simulink model "untitled"  (R2025b)
settings: Solver=FixedStepAuto  StartTime=0.0  StopTime=20  FixedStep=0.001  RelTol=1e-3
libraries: simulink x2, slpidlib x2
settings Model: Creator=Utente  LastModifiedBy=zinga

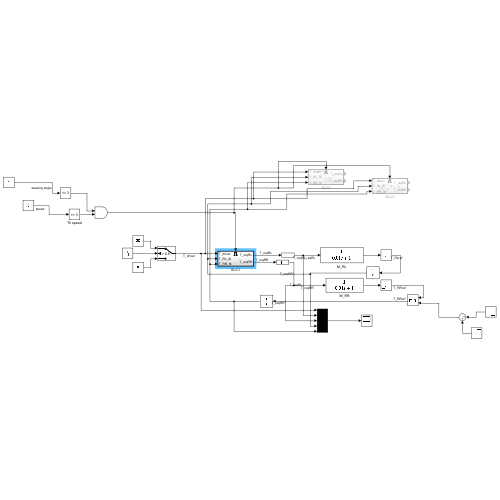
[thumbnail: Simulink's stored preview of the top-level diagram]
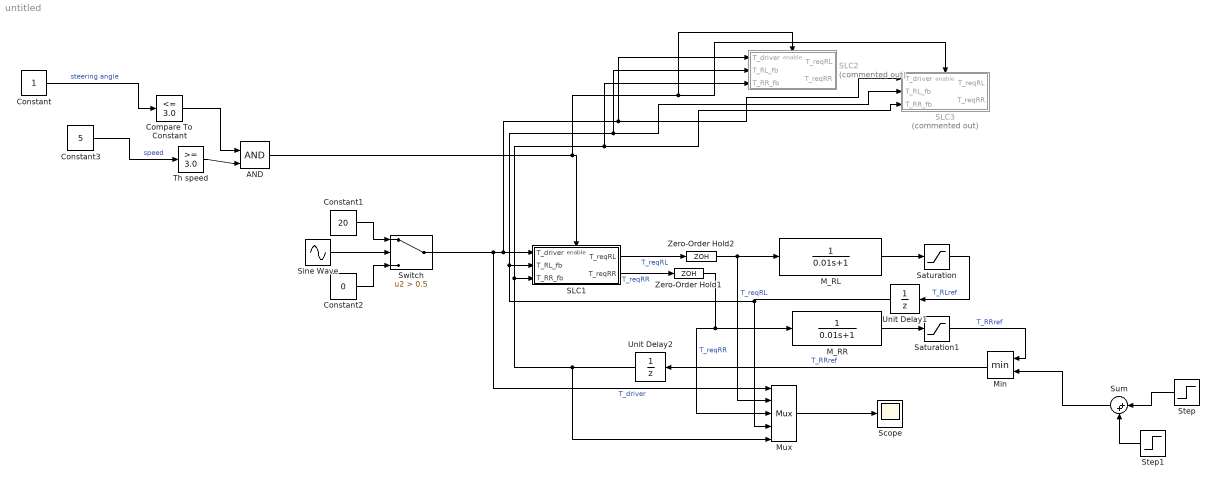
== system untitled ==
  AND : Logic  IconShape=distinctive  AllPortsSameDT=off  OutDataTypeStr=boolean
  Compare To Constant : simulink/Logic and Bit Operations/Compare To Constant  relop=<=  const=3.0  OutDataTypeStr=boolean
  Constant : Constant
  Constant1 : Constant  Value=20
  Constant2 : Constant  Value=0
  Constant3 : Constant  Value=5
  M_RL : TransferFcn  Denominator=[0.01 1]
  M_RR : TransferFcn  Denominator=[0.01 1]
  Min : MinMax  Inputs=2
  Mux : Mux  Inputs=5
  SLC1 : Subsystem  TreatAsAtomicUnit=on
  SLC2 : Subsystem  Commented=on  TreatAsAtomicUnit=on
  SLC3 : Subsystem  Commented=on  TreatAsAtomicUnit=on
  Saturation : Saturate  UpperLimit=21  LowerLimit=-21
  Saturation1 : Saturate  UpperLimit=21  LowerLimit=-21
  Scope : Scope
      settings: ActiveDisplayYMinimum=1.4080718802065189  ActiveDisplayYMaximum=18.911191161536266
  Sine Wave : Sin  Frequency=0.2  SampleTime=0.01
  Step : Step  Time=3  Before=21  After=8  SampleTime=0
  Step1 : Step  Time=9  After=13  SampleTime=0
  Sum : Sum  Inputs=|++
  Switch : Switch  Criteria=u2 > Threshold  Threshold=0.5  SaturateOnIntegerOverflow=off  InputSameDT=off
  Th speed : simulink/Logic and Bit Operations/Compare To Constant  relop=>=  const=3.0  OutDataTypeStr=boolean
  Unit Delay1 : UnitDelay  SampleTime=-1  HasFrameUpgradeWarning=on
  Unit Delay2 : UnitDelay  SampleTime=-1  HasFrameUpgradeWarning=on
  Zero-Order Hold1 : ZeroOrderHold  SampleTime=0.01
  Zero-Order Hold2 : ZeroOrderHold  SampleTime=0.01
  wires:
  Compare To Constant/1 -> AND/1
  Constant/1 -> Compare To Constant/1  "steering angle"
  SLC1/1(T_reqRL) -> Zero-Order Hold2/1  "T_reqRL"
  SLC1/2(T_reqRR) -> Zero-Order Hold1/1  "T_reqRR"
  Mux/1 -> Scope/1
  M_RL/1 -> Saturation/1
  Saturation/1 -> Unit Delay1/1  "T_RLref"
  Sine Wave/1 -> Switch/2
  Constant1/1 -> Switch/1
  Constant2/1 -> Switch/3
  Switch/1 -> Mux/1, SLC3/1(T_driver), SLC2/1(T_driver), SLC1/1(T_driver)  "T_driver"
  M_RR/1 -> Saturation1/1
  Min/1 -> Unit Delay2/1  "T_RRref"
  Constant3/1 -> Th speed/1  "speed"
  Th speed/1 -> AND/2
  AND/1 -> SLC1/Enable, SLC3/Enable, SLC2/Enable
  Saturation1/1 -> Min/1  "T_RRref"
  Step/1 -> Sum/1
  Sum/1 -> Min/2
  Step1/1 -> Sum/2
  Unit Delay1/1 -> Mux/4, SLC1/2(T_RL_fb), SLC3/2(T_RL_fb), SLC2/2(T_RL_fb)
  Unit Delay2/1 -> SLC2/3(T_RR_fb), SLC3/3(T_RR_fb), SLC1/3(T_RR_fb), Mux/5
  Zero-Order Hold1/1 -> Mux/3, M_RR/1  "T_reqRR"
  Zero-Order Hold2/1 -> Mux/2, M_RL/1  "T_reqRL"

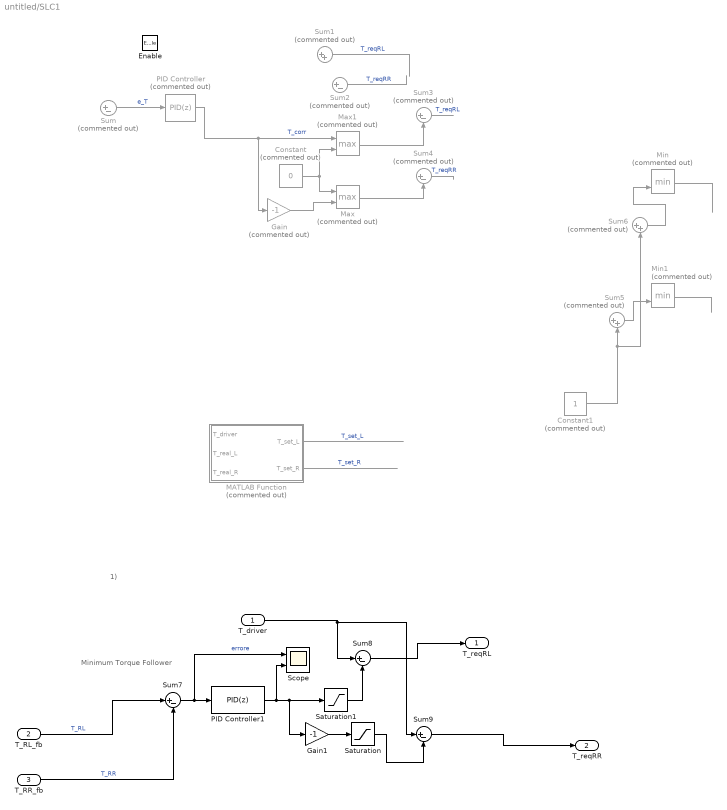
== system untitled/SLC1 ==
  note: Minimum Torque Follower
  note: 1)
  T_driver : Inport
  T_RL_fb : Inport  Port=2
  T_RR_fb : Inport  Port=3
  Enable : EnablePort
  Constant : Constant  Commented=on  Value=0
  Constant1 : Constant  Commented=on
  Gain : Gain  Commented=on  Gain=-1
  Gain1 : Gain  Gain=-1
  MATLAB Function : MATLAB Function  Commented=on  TreatAsAtomicUnit=on
  Max : MinMax  Commented=on  Function=max  Inputs=2
  Max1 : MinMax  Commented=on  Function=max  Inputs=2
  Min : MinMax  Commented=on  Inputs=2
  Min1 : MinMax  Commented=on  Inputs=2
  PID Controller : slpidlib/PID Controller  Commented=on  Controller=PID  Form=Parallel  TimeDomain=Discrete-time  UseExternalTs=off  SampleTime=0.05  IntegratorMethod=Forward Euler  FilterMethod=Forward Euler  ControllerParametersSource=internal  P=0.02  I=5  UseKiTs=off  D=0  UseExternalDerivativeSource=off  N=100  UseFilter=on  TunerSelectOption=Transfer Function Based (PID Tuner App)  InitialConditionSource=internal  InitialConditionForIntegrator=0  InitialConditionForFilter=0  DifferentiatorICPrevScaledInput=0  ExternalReset=none  TrackingMode=off  Kt=1  LimitOutput=on  SatLimitsSource=internal  UpperSaturationLimit=21  LowerSaturationLimit=-21  LinearizeAsGain=on  AntiWindupMode=clamping  Kb=1  LimitIntegrator=off  UpperIntegratorSaturationLimit=inf  LowerIntegratorSaturationLimit=-inf  POutMin=[]  POutMax=[]  IOutMin=[]  IOutMax=[]  DOutMin=[]  DOutMax=[]  NOutMin=[]  NOutMax=[]  SumOutMin=[]  SumOutMax=[]  SaturationOutMin=[]  SaturationOutMax=[]  PParamMin=[]  PParamMax=[]  IParamMin=[]  IParamMax=[]  DParamMin=[]  DParamMax=[]  NParamMin=[]  NParamMax=[]  KbParamMin=[]  KbParamMax=[]  KtParamMin=[]  KtParamMax=[]  KbOutMin=[]  KbOutMax=[]  KtOutMin=[]  KtOutMax=[]  IntegratorOutMin=[]  IntegratorOutMax=[]  FilterOutMin=[]  FilterOutMax=[]  SumI1OutMin=[]  SumI1OutMax=[]  SumI2OutMin=[]  SumI2OutMax=[]  SumI3OutMin=[]  SumI3OutMax=[]  SumI4OutMin=[]  SumI4OutMax=[]  SumDOutMin=[]  SumDOutMax=[]  DifferentiatorOutMin=[]  DifferentiatorOutMax=[]  FilterDiffOutCoefMin=[]  FilterDiffOutCoefMax=[]  ReciprocalOutMin=[]  ReciprocalOutMax=[]  SumDenOutMin=[]  SumDenOutMax=[]  SumNumOutMin=[]  SumNumOutMax=[]  DivideOutMin=[]  DivideOutMax=[]  UdiffTsProdOutMin=[]  UdiffTsProdOutMax=[]  NTsProdOutMin=[]  NTsProdOutMax=[]  UintegralTsProdOutMin=[]  UintegralTsProdOutMax=[]  UngainTsProdOutMin=[]  UngainTsProdOutMax=[]  ClampingZeroOutDataTypeStr=Inherit: Inherit via back propagation  ClampingZeroOutMin=[]  ClampingZeroOutMax=[]  FilterDenConstantOutDataTypeStr=Inherit: Inherit via back propagation  FilterDenConstantOutMin=[]  FilterDenConstantOutMax=[]  PCopyOutDataTypeStr=Inherit: Inherit via back propagation  PCopyOutMin=[]  PCopyOutMax=[]  NCopyOutDataTypeStr=Inherit: Inherit via back propagation  NCopyOutMin=[]  NCopyOutMax=[]  IntegratorContinuousStateAttributes=''  IntegratorStateMustResolveToSignalObject=off  IntegratorRTWStateStorageClass=Auto  FilterContinuousStateAttributes=''  FilterStateMustResolveToSignalObject=off  FilterRTWStateStorageClass=Auto  ParallelPVariant=InternalParameters  IdealPVariant=Disabled  IVariant=InternalParameters  DVariant=InternalParameters  IntegratorVariant=Discrete  SatVariant=Enabled  AWVariant=DiscClampingParallel  PCopyVariant=Disabled  TRVariant=Disabled  FdbkBlocksVariant=Forward  IdealPFdbkVariant=Disabled  SatFdbkVariant=Disabled  DerivativeFilterVariant=ForwardEulerFilter  NVariant=InternalParameters  NCopyVariant=Disabled  FilterICVariant=InternalICsFilter  IntegratorICVariant=InternalICs  ExternalResetVariant=Disabled  TRSumVariant=Passthrough  SumFdbkVariant=Disabled  SumVariant=Sum_PID  TsampFilterVariant=InternalTs  TsampNgainVariant=Passthrough  TsampIntegralVariant=Disabled_SignalSpec  ExternalSaturationOutDataTypeStr=Inherit: Same as second input  DerivativeSourceVariant=ErrorSignal  PreIntVariant=InternalPreInt
  PID Controller1 : slpidlib/PID Controller  Controller=PID  Form=Parallel  TimeDomain=Discrete-time  UseExternalTs=off  SampleTime=0.01  IntegratorMethod=Forward Euler  FilterMethod=Forward Euler  ControllerParametersSource=internal  P=0.735101548489  I=1.708978857120148  UseKiTs=off  D=0  UseExternalDerivativeSource=off  N=100  UseFilter=off  TunerSelectOption=Transfer Function Based (PID Tuner App)  InitialConditionSource=internal  InitialConditionForIntegrator=0  InitialConditionForFilter=0  DifferentiatorICPrevScaledInput=0  ExternalReset=none  TrackingMode=off  Kt=1  LimitOutput=on  SatLimitsSource=internal  UpperSaturationLimit=17  LowerSaturationLimit=-17  LinearizeAsGain=on  AntiWindupMode=clamping  Kb=1  LimitIntegrator=off  UpperIntegratorSaturationLimit=inf  LowerIntegratorSaturationLimit=-inf  POutMin=[]  POutMax=[]  IOutMin=[]  IOutMax=[]  DOutMin=[]  DOutMax=[]  NOutMin=[]  NOutMax=[]  SumOutMin=[]  SumOutMax=[]  SaturationOutMin=[]  SaturationOutMax=[]  PParamMin=[]  PParamMax=[]  IParamMin=[]  IParamMax=[]  DParamMin=[]  DParamMax=[]  NParamMin=[]  NParamMax=[]  KbParamMin=[]  KbParamMax=[]  KtParamMin=[]  KtParamMax=[]  KbOutMin=[]  KbOutMax=[]  KtOutMin=[]  KtOutMax=[]  IntegratorOutMin=[]  IntegratorOutMax=[]  FilterOutMin=[]  FilterOutMax=[]  SumI1OutMin=[]  SumI1OutMax=[]  SumI2OutMin=[]  SumI2OutMax=[]  SumI3OutMin=[]  SumI3OutMax=[]  SumI4OutMin=[]  SumI4OutMax=[]  SumDOutMin=[]  SumDOutMax=[]  DifferentiatorOutMin=[]  DifferentiatorOutMax=[]  FilterDiffOutCoefMin=[]  FilterDiffOutCoefMax=[]  ReciprocalOutMin=[]  ReciprocalOutMax=[]  SumDenOutMin=[]  SumDenOutMax=[]  SumNumOutMin=[]  SumNumOutMax=[]  DivideOutMin=[]  DivideOutMax=[]  UdiffTsProdOutMin=[]  UdiffTsProdOutMax=[]  NTsProdOutMin=[]  NTsProdOutMax=[]  UintegralTsProdOutMin=[]  UintegralTsProdOutMax=[]  UngainTsProdOutMin=[]  UngainTsProdOutMax=[]  ClampingZeroOutDataTypeStr=Inherit: Inherit via back propagation  ClampingZeroOutMin=[]  ClampingZeroOutMax=[]  FilterDenConstantOutDataTypeStr=Inherit: Inherit via back propagation  FilterDenConstantOutMin=[]  FilterDenConstantOutMax=[]  PCopyOutDataTypeStr=Inherit: Inherit via back propagation  PCopyOutMin=[]  PCopyOutMax=[]  NCopyOutDataTypeStr=Inherit: Inherit via back propagation  NCopyOutMin=[]  NCopyOutMax=[]  IntegratorContinuousStateAttributes=''  IntegratorStateMustResolveToSignalObject=off  IntegratorRTWStateStorageClass=Auto  FilterContinuousStateAttributes=''  FilterStateMustResolveToSignalObject=off  FilterRTWStateStorageClass=Auto  ParallelPVariant=InternalParameters  IdealPVariant=Disabled  IVariant=InternalParameters  DVariant=InternalParameters  IntegratorVariant=Discrete  SatVariant=Enabled  AWVariant=DiscClampingParallel  PCopyVariant=Disabled  TRVariant=Disabled  FdbkBlocksVariant=Forward  IdealPFdbkVariant=Disabled  SatFdbkVariant=Disabled  DerivativeFilterVariant=Differentiator  NVariant=Passthrough  NCopyVariant=Disabled_SignalSpec  FilterICVariant=InternalICsDifferentiator  IntegratorICVariant=InternalICs  ExternalResetVariant=Disabled  TRSumVariant=Passthrough  SumFdbkVariant=Disabled  SumVariant=Sum_PID  TsampFilterVariant=InternalTs  TsampNgainVariant=Passthrough  TsampIntegralVariant=Disabled_SignalSpec  ExternalSaturationOutDataTypeStr=Inherit: Same as second input  DerivativeSourceVariant=ErrorSignal  PreIntVariant=InternalPreInt
  Saturation : Saturate  UpperLimit=inf  LowerLimit=0
  Saturation1 : Saturate  UpperLimit=inf  LowerLimit=0
  Scope : Scope  NumInputPorts=2
      settings: ActiveDisplayYMinimum=-14.99995177507224  ActiveDisplayYMaximum=14.999994641674681
  Sum{,2..4} (4 alike) : Sum  Commented=on  Inputs=|+-
  Sum1 : Sum  Commented=on  Inputs=|++
  Sum5 : Sum  Commented=on  Inputs=|++
  Sum6 : Sum  Commented=on  Inputs=|++
  Sum7 : Sum  Inputs=|+-
  Sum8 : Sum  Inputs=|+-
  Sum9 : Sum  Inputs=|+-
  T_reqRL : Outport
  T_reqRR : Outport  Port=2
  wires:
  ? -> MATLAB Function/3(T_real_R), Sum6/1, Sum/2  "T_RR"
  ? -> MATLAB Function/2(T_real_L), Sum5/1, Sum/1  "T_RL"
  Sum/1 -> PID Controller/1  "e_T"
  Sum2/1 -> ?  "T_reqRR"
  Sum1/1 -> ?  "T_reqRL"
  ? -> Min1/1, Min/1, MATLAB Function/1(T_driver), Sum4/1, Sum3/1, Sum2/1, Sum1/1  "T_driver"
  MATLAB Function/1(T_set_L) -> ?  "T_set_L"
  MATLAB Function/2(T_set_R) -> ?  "T_set_R"
  Constant/1 -> Max/1, Max1/2
  PID Controller/1 -> Gain/1, Max1/1  "T_corr"
  Gain/1 -> Max/2
  Max/1 -> Sum4/2
  Max1/1 -> Sum3/2
  Sum3/1 -> ?  "T_reqRL"
  Sum4/1 -> ?  "T_reqRR"
  Min1/1 -> ?
  Min/1 -> ?
  Constant1/1 -> Sum6/2, Sum5/2
  Sum5/1 -> Min1/2
  Sum6/1 -> Min/2
  T_RL_fb/1 -> Sum7/1  "T_RL"
  T_RR_fb/1 -> Sum7/2  "T_RR"
  T_driver/1 -> Sum9/1, Sum8/1
  PID Controller1/1 -> Saturation1/1, Gain1/1, Scope/2
  Sum8/1 -> T_reqRL/1
  Gain1/1 -> Saturation/1
  Saturation/1 -> Sum9/2
  Sum9/1 -> T_reqRR/1
  Saturation1/1 -> Sum8/2
  Sum7/1 -> Scope/1, PID Controller1/1  "errore"

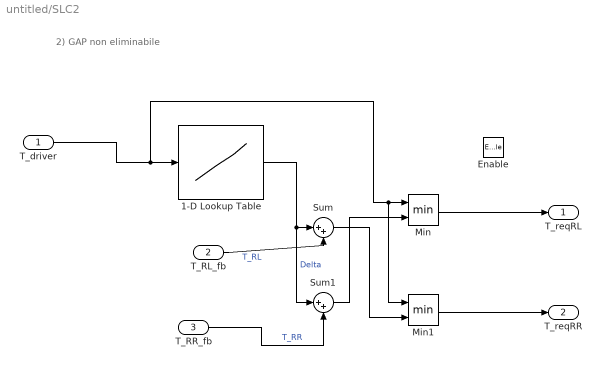
== system untitled/SLC2 ==
  note: 2) GAP non eliminabile
  T_driver : Inport
  T_RL_fb : Inport  Port=2
  T_RR_fb : Inport  Port=3
  Enable : EnablePort
  1-D Lookup Table : Lookup_n-D  NumberOfTableDimensions=1  BreakpointsForDimension1=[0 5 10 15 21]  Table=[5 3 2 1 1]  InternalRulePriority=Speed  RndMeth=Simplest
  Min : MinMax  Inputs=2
  Min1 : MinMax  Inputs=2
  Sum : Sum  Inputs=|++
  Sum1 : Sum  Inputs=|++
  T_reqRL : Outport
  T_reqRR : Outport  Port=2
  wires:
  T_driver/1 -> Min1/1, Min/1, 1-D Lookup Table/1
  Min1/1 -> T_reqRR/1
  Min/1 -> T_reqRL/1
  1-D Lookup Table/1 -> Sum1/1, Sum/1  "Delta"
  T_RL_fb/1 -> Sum/2  "T_RL"
  T_RR_fb/1 -> Sum1/2  "T_RR"
  Sum/1 -> Min1/2
  Sum1/1 -> Min/2

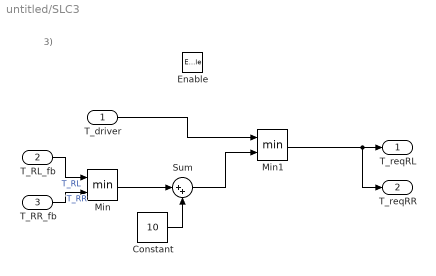
== system untitled/SLC3 ==
  note: 3)
  T_driver : Inport
  T_RL_fb : Inport  Port=2
  T_RR_fb : Inport  Port=3
  Enable : EnablePort
  Constant : Constant  Value=10
  Min : MinMax  Inputs=2
  Min1 : MinMax  Inputs=2
  Sum : Sum  Inputs=|++
  T_reqRL : Outport
  T_reqRR : Outport  Port=2
  wires:
  T_RL_fb/1 -> Min/1  "T_RL"
  T_RR_fb/1 -> Min/2  "T_RR"
  Min/1 -> Sum/1
  Constant/1 -> Sum/2
  T_driver/1 -> Min1/1
  Sum/1 -> Min1/2
  Min1/1 -> T_reqRR/1, T_reqRL/1

== matlab function untitled/SLC1/MATLAB Function ==
  data: T_driver input; T_set_L output; T_real_L input; T_real_R input; T_set_R output
function [T_set_L, T_set_R] = fcn(T_driver, T_real_L, T_real_R)

    % Imposta una tolleranza 0.1Nm per ignorare il rumore
    tolleranza = 0.1; 
    
    % Calcola la differenza assoluta tra le due ruote
    delta_T = abs(T_real_L - T_real_R);
    
    if delta_T <= tolleranza
        % Tutto ok (inclusa partenza da fermo e coasting)
        T_set_L = T_driver;
        T_set_R = T_driver;
    else
        % Un motore è in derating termico/meccanico. 
        if T_real_L < T_real_R
            % Il sinistro è in crisi
            T_set_L = T_driver; 
            T_set_R = T_real_L; 
        else
            % Il destro è in crisi
            T_set_L = T_real_R; 
            T_set_R = T_driver; 
        end
    end
end
